simulink model "STH_NL"  (R2020b)
settings: Solver=FixedStepAuto  StartTime=0.0  StopTime=1800  FixedStep=5  RelTol=1e-3
values from neighbouring files (symbols this model uses):
  Fjs = 7.079e-4    (= 0.0007079)    [Exp3_STH.m]
  Fs = 4.720e-4    (= 0.000472)    [Exp3_STH.m]
  Tis = 10    [Exp3_STH.m]
  Tjis = 93.33    [Exp3_STH.m]
  Tjs = 65.56    [Exp3_STH.m]
  Ts = 51.67    [Exp3_STH.m]
settings Model: Creator=franc  LastModifiedBy=franc

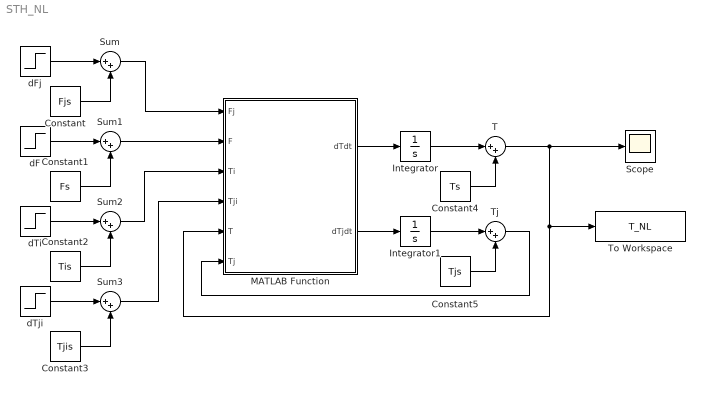
== system STH_NL ==
  "            T" : Sum  Inputs=|++
  "            Tj" : Sum  Inputs=|++
  Constant : Constant  Value=Fjs
  Constant1 : Constant  Value=Fs
  Constant2 : Constant  Value=Tis
  Constant3 : Constant  Value=Tjis
  Constant4 : Constant  Value=Ts
  Constant5 : Constant  Value=Tjs
  Integrator : Integrator
  Integrator1 : Integrator
  MATLAB Function : MATLAB Function  TreatAsAtomicUnit=on
  Scope : Scope
  Sum{,1..3} (4 alike) : Sum  Inputs=|++
  To Workspace : ToWorkspace  VariableName=T_NL  SaveFormat=Timeseries  SampleTime=-1
  dF : Step  Time=0  After=0  SampleTime=0
  dFj : Step  Time=0  After=4.72e-5  SampleTime=0
  dTi : Step  Time=0  After=0  SampleTime=0
  dTji : Step  Time=0  After=0  SampleTime=0
  wires:
  Constant2/1 -> Sum2/2
  Sum/1 -> MATLAB Function/1(Fj)
  Sum3/1 -> MATLAB Function/4(Tji)
  dF/1 -> Sum1/1
  Constant1/1 -> Sum1/2
  Sum2/1 -> MATLAB Function/3(Ti)
  dTji/1 -> Sum3/1
  dFj/1 -> Sum/1
  Constant3/1 -> Sum3/2
  dTi/1 -> Sum2/1
  Constant/1 -> Sum/2
  Sum1/1 -> MATLAB Function/2(F)
  MATLAB Function/1(dTdt) -> Integrator/1
  MATLAB Function/2(dTjdt) -> Integrator1/1
  Integrator/1 -> "            T"/1
  Constant4/1 -> "            T"/2
  Constant5/1 -> "            Tj"/2
  Integrator1/1 -> "            Tj"/1
  "            Tj"/1 -> MATLAB Function/6(Tj)
  "            T"/1 -> Scope/1, MATLAB Function/5(T), To Workspace/1

== matlab function STH_NL/MATLAB Function ==
  data: Fj input; dTdt output; dTjdt output; F input; Ti input; Tji input; T input; Tj input
function [dTdt, dTjdt] = fcn(Fj, F, Ti, Tji, T, Tj)
% Definição dos parâmetros da simulação
V      = 283.168e-3; % Volume do tanque [m^3]
Vj     = 28.319e-3;  % Volume da jaqueta [m^3]
rhocp  = 2.165e3;    % Densidade*Cap. calorífica do fluido no tanque [W/(ºC*m^3)]
rhocpj = 2.165e3;    % Densidade*Cap. calorífica do fluido na jaqueta [W/(ºC*m^3)]
UA     = 3.065;      % Coef. de transf. de calor*Área da superfície [W/(ºC*min)]

% Equação diferencial que descreve ocomportamento dinâmico da temperatura:
dTdt  = F/V*(Ti - T) + (UA*(Tj - T))/(V*rhocp);

% Equação diferencial para a temperatura do fluido na jaqueta:
dTjdt = Fj/Vj*(Tji - Tj) - (UA*(Tj - T))/(Vj*rhocpj);
